simulink model "es2sim"  (R2023b)
settings: Solver=VariableStepAuto  StartTime=0.0  StopTime=Tfin  RelTol=1e-3
values from neighbouring files (symbols this model uses):
  beta0 = [0 0 0]'    [es2.m]    (also in es3.m)
  IJ = inv(J)    [es1.m]    (also in es2.m; es3.m)
  J = [937.5 833.3 270.8]    [dyn_kin_quat.m]    (also in es1.m = diag([937.5, 833.3, 270.8]); es2.m = diag([937.5, 833.3, 270.8]); es3.m = diag([937.5, 833.3, 270.8]); euler_eq.m = [400 50 150])
  M = [0,0,0]'    [es1.m]    (also in es2.m = [0 0 0]; es3.m = [0 0 0])
  w0 = [1,0.1,0]'    [es1.m]    (also in es2.m; es3.m)
libraries: vrlib x1
settings Model: Creator=luigi  LastModifiedBy=luigi

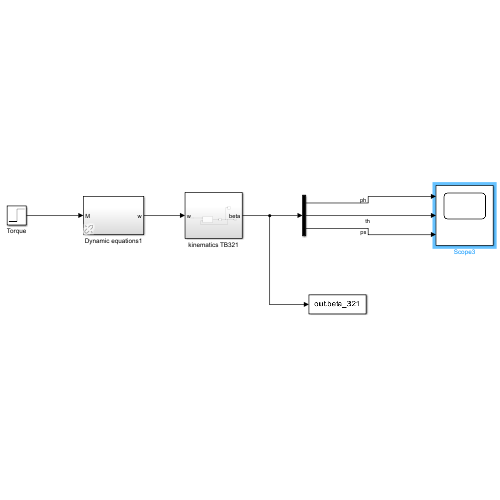
[thumbnail: Simulink's stored preview of the top-level diagram]
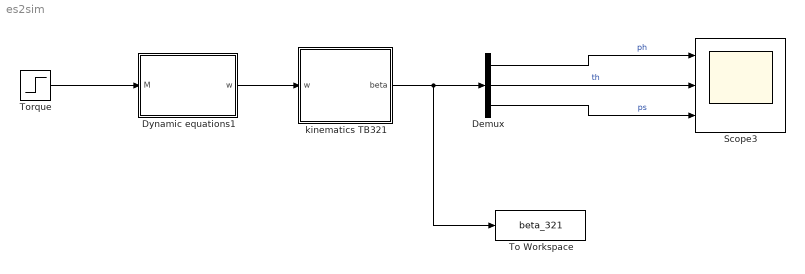
== system es2sim ==
  Demux : Demux  Outputs=3
  Dynamic equations1 : Subsystem  AncestorBlock=lib_rotations_2014/Euler equation
  Scope3 : Scope  NumInputPorts=3
  To Workspace : ToWorkspace  VariableName=beta_321  SaveFormat=Timeseries  SampleTime=-1
  Torque : Step  Time=0  After=M  SampleTime=0
  kinematics TB321 : Subsystem
  wires:
  Dynamic equations1/1(w) -> kinematics TB321/1(w)
  Torque/1 -> Dynamic equations1/1(M)
  Demux/2 -> Scope3/2  "th"
  kinematics TB321/1(beta) -> Demux/1, To Workspace/1
  Demux/3 -> Scope3/3  "ps"
  Demux/1 -> Scope3/1  "ph"

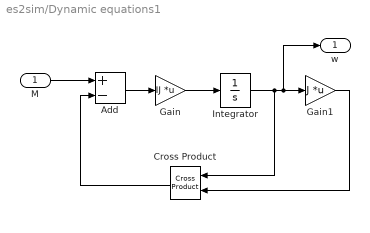
== system es2sim/Dynamic equations1 ==
  M : Inport
  Add : Sum  Inputs=+-
  Cross Product : vrlib/Utilities/Cross Product
  Gain : Gain  Gain=IJ  Multiplication=Matrix(K*u)
  Gain1 : Gain  Gain=J  Multiplication=Matrix(K*u)
  Integrator : Integrator  InitialCondition=w0
  w : Outport  VectorParamsAs1DForOutWhenUnconnected=off
  wires:
  Cross Product/1 -> Add/2
  Add/1 -> Gain/1
  Gain1/1 -> Cross Product/2
  Gain/1 -> Integrator/1
  Integrator/1 -> Gain1/1, w/1, Cross Product/1
  M/1 -> Add/1

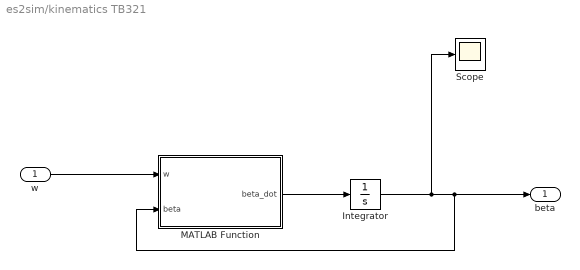
== system es2sim/kinematics TB321 ==
  w : Inport  PortDimensions=3
  Integrator : Integrator  InitialCondition=beta0
  MATLAB Function : MATLAB Function  TreatAsAtomicUnit=on
  Scope : Scope
  beta : Outport  PortDimensions=3  VectorParamsAs1DForOutWhenUnconnected=off
  wires:
  w/1 -> MATLAB Function/1(w)
  MATLAB Function/1(beta_dot) -> Integrator/1
  Integrator/1 -> beta/1, MATLAB Function/2(beta), Scope/1

== matlab function es2sim/kinematics TB321/MATLAB Function ==
  data: w input; beta_dot output; beta input
function beta_dot = kinTB_321(w,beta)
%The function kinTB_321(w,beta) compute the kinematics of TB-321 using the
%inverse of the DCM matrix. The parametres are omega, the angular velocity,
%and angles.

ph = beta(1);
th = beta(2);
ps = beta(3);

T = [cos(th) sin(ph)*sin(th) cos(ph)*sin(th);
       0 cos(ph)*cos(th) -cos(th)*sin(ph);
       0         sin(ph)          cos(ph)];
T = T/cos(th);
   
beta_dot = T*w;

end
